simulink model "Batteri_Transducers_1I_1U"  (R2020b)
settings: Solver=VariableStepAuto  StartTime=0.0  StopTime=0.01  RelTol=1e-3
libraries: fl_lib x26, nesl_utility x10, ee_lib x2
settings Model: Creator=jenel  LastModifiedBy=jenel

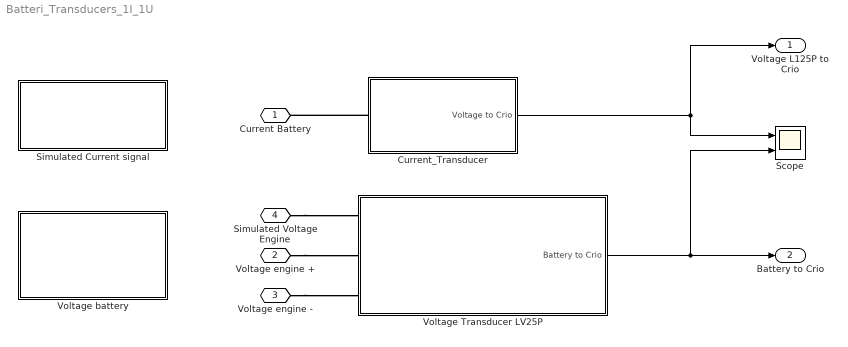
== system Batteri_Transducers_1I_1U ==
  Current_Transducer : Subsystem
  Scope : Scope  NumInputPorts=2
  Simulated Current signal : Subsystem
  Voltage Transducer LV25P : Subsystem
  Voltage battery : Subsystem
  Current Battery : PMIOPort  Side=Left
  Voltage engine + : PMIOPort  Port=2  Side=Left
  Voltage engine - : PMIOPort  Port=3  Side=Left
  Simulated Voltage Engine : PMIOPort  Port=4  Side=Right
  "Voltage L125P to Crio " : Outport
  Battery to Crio : Outport  Port=2
  wires:
  Voltage Transducer LV25P/1(Battery to Crio) -> Scope/2, Battery to Crio/1
  Current_Transducer/1(Voltage to Crio) -> Scope/1, "Voltage L125P to Crio "/1
  connections:
  Simulated Voltage Engine/RConn1 -- Voltage Transducer LV25P/LConn1
  Voltage engine +/RConn1 -- Voltage Transducer LV25P/LConn2
  Voltage engine -/RConn1 -- Voltage Transducer LV25P/LConn3
  Current_Transducer/LConn1 -- Current Battery/RConn1

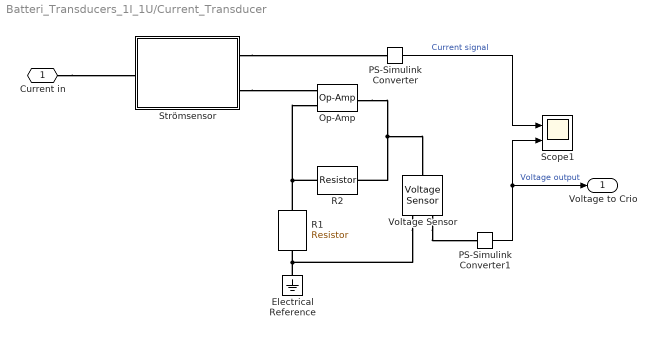
== system Batteri_Transducers_1I_1U/Current_Transducer ==
  Electrical Reference : fl_lib/Electrical/Electrical Elements/Electrical Reference
  Op-Amp : fl_lib/Electrical/Electrical Elements/Op-Amp  outI_specify=on  outI_priority=None  outI=0 A  outI_nominal_specify=off  outI_nominal_unit=A  outI_nominal_value=1
  PS-Simulink Converter : nesl_utility/PS-Simulink Converter  PhysicalDomain=network_engine_domain  SubClassName=ps_output  LeftPortType=input  RightPortType=output  PseudoPeriodic=off  Frequencies=[]  Unit=inherit  AffineConversion=off
  PS-Simulink Converter1 : nesl_utility/PS-Simulink Converter  PhysicalDomain=network_engine_domain  SubClassName=ps_output  LeftPortType=input  RightPortType=output  PseudoPeriodic=off  Frequencies=[]  Unit=inherit  AffineConversion=off
  R1 : fl_lib/Electrical/Electrical Elements/Resistor  R=1000 Ohm  i_specify=off  i_priority=None  i=0 A  i_nominal_specify=off  i_nominal_unit=A  i_nominal_value=1  v_specify=off  v_priority=None  v=0 V  v_nominal_specify=off  v_nominal_unit=V  v_nominal_value=1
  R2 : fl_lib/Electrical/Electrical Elements/Resistor  R=666.6667 Ohm  i_specify=off  i_priority=None  i=0 A  i_nominal_specify=off  i_nominal_unit=A  i_nominal_value=1  v_specify=off  v_priority=None  v=0 V  v_nominal_specify=off  v_nominal_unit=V  v_nominal_value=1
  Scope1 : Scope  NumInputPorts=2
  Strömsensor : Subsystem
  Voltage Sensor : fl_lib/Electrical/Electrical Sensors/Voltage Sensor
  Current in : PMIOPort  Side=Left
  Voltage to Crio : Outport
  wires:
  PS-Simulink Converter1/1 -> Scope1/2, Voltage to Crio/1  "Voltage output"
  PS-Simulink Converter/1 -> Scope1/1  "Current signal"
  connections:
  Strömsensor/RConn2 -- Op-Amp/LConn1
  R2/LConn1 -- R1/LConn1 -- Op-Amp/LConn2
  Current in/RConn1 -- Strömsensor/LConn1
  Strömsensor/RConn1 -- PS-Simulink Converter/LConn1
  Op-Amp/RConn1 -- Voltage Sensor/LConn1 -- R2/RConn1
  Electrical Reference/LConn1 -- R1/RConn1 -- Voltage Sensor/RConn2
  Voltage Sensor/RConn1 -- PS-Simulink Converter1/LConn1

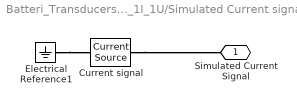
== system Batteri_Transducers_1I_1U/Simulated Current signal ==
  Current signal : ee_lib/Sources/Current Source  dc_current=200 mA  ac_current=0 mA  ac_shift=0 rad  ac_frequency=0 Hz  noise_mode=0  PSD=0 A^2/Hz  repeatability=1  auto_seed=153380492  user_seed=0  sample_time=1e-3 s  i_specify=off  i_priority=None  i=0 A  i_nominal_specify=off  i_nominal_unit=A  i_nominal_value=1  v_specify=off  v_priority=None  v=0 V  v_nominal_specify=off  v_nominal_unit=V  v_nominal_value=1
      settings: SourceProductBaseCode=PS
  Electrical Reference1 : fl_lib/Electrical/Electrical Elements/Electrical Reference
  Simulated Current Signal : PMIOPort  Side=Right
  connections:
  Electrical Reference1/LConn1 -- Current signal/RConn1
  Current signal/LConn1 -- Simulated Current Signal/RConn1

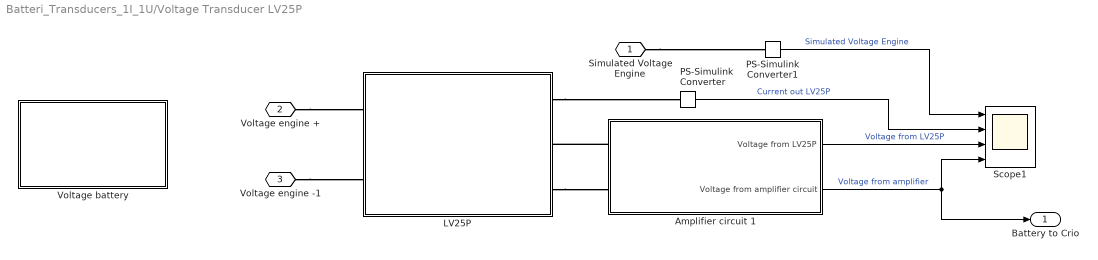
== system Batteri_Transducers_1I_1U/Voltage Transducer LV25P ==
  Amplifier circuit 1 : Subsystem
  LV25P : Subsystem
  PS-Simulink Converter : nesl_utility/PS-Simulink Converter  PhysicalDomain=network_engine_domain  SubClassName=ps_output  LeftPortType=input  RightPortType=output  PseudoPeriodic=off  Frequencies=[]  Unit=inherit  AffineConversion=off
  PS-Simulink Converter1 : nesl_utility/PS-Simulink Converter  PhysicalDomain=network_engine_domain  SubClassName=ps_output  LeftPortType=input  RightPortType=output  PseudoPeriodic=off  Frequencies=[]  Unit=inherit  AffineConversion=off
  Scope1 : Scope  NumInputPorts=4
  Voltage battery : Subsystem
  Simulated Voltage Engine : PMIOPort  Side=Left
  Voltage engine + : PMIOPort  Port=2  Side=Left
  Voltage engine -1 : PMIOPort  Port=3  Side=Left
  Battery to Crio : Outport
  wires:
  Amplifier circuit 1/1(Voltage from LV25P) -> Scope1/3  "Voltage from LV25P"
  PS-Simulink Converter1/1 -> Scope1/1  "Simulated Voltage Engine"
  Amplifier circuit 1/2(Voltage from amplifier circuit) -> Scope1/4, Battery to Crio/1  "Voltage from amplifier"
  PS-Simulink Converter/1 -> Scope1/2  "Current out LV25P"
  connections:
  Voltage engine +/RConn1 -- LV25P/LConn1
  Simulated Voltage Engine/RConn1 -- PS-Simulink Converter1/LConn1
  Amplifier circuit 1/LConn1 -- LV25P/RConn2
  LV25P/RConn1 -- PS-Simulink Converter/LConn1
  LV25P/RConn3 -- Amplifier circuit 1/LConn2
  Voltage engine -1/RConn1 -- LV25P/LConn2

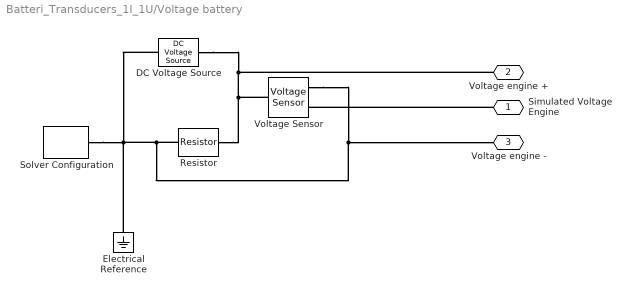
== system Batteri_Transducers_1I_1U/Voltage battery ==
  DC Voltage Source : ee_lib/Additional Components/SPICE Sources/DC Voltage Source  DC=144 V
  Electrical Reference : fl_lib/Electrical/Electrical Elements/Electrical Reference
  Resistor : fl_lib/Electrical/Electrical Elements/Resistor  R=10 Ohm  i_specify=off  i_priority=None  i=0 A  i_nominal_specify=off  i_nominal_unit=A  i_nominal_value=1  v_specify=off  v_priority=None  v=0 V  v_nominal_specify=off  v_nominal_unit=V  v_nominal_value=1
  Solver Configuration : nesl_utility/Solver Configuration  PhysicalDomain=network_engine_domain  SubClassName=solver  LeftPortType=input  RightPortType=generic  Tones=[]  Harmonics=[]  SimulateNoise=off  Profile=off  UseLocalSampling=off  EnableSwitchedLinearOptims=on  FrequencyDomain=off  UseCCode=off  RelTol=0.001  AbsTol=1e-06  MinStep=1e-09  ToWorkspace=off  RevertToSquareIcSolve=off  NumHomotopyIterations=100  PhasorMode=off  PhasorModeNumHarmonics=1  DoDC=off  ResidualTolerance=1e-09  UseLocalSolver=off  LocalSolverChoice=NE_BACKWARD_EULER_ADVANCER  LocalSolverSampleTime=0.001  DoFixedCost=off  MaxNonlinIter=3  MaxModeIter=2  ComputeImpulses=off  ImpulseIterations=2  LinearAlgebra=auto  EquationFormulation=NE_TIME_EF  DelaysMemoryBudget=1024  AutomaticFiltering=on  FilteringTimeConstant=0.001  PartitionStorageMethod=AS_NEEDED  PartitionMemoryBudget=1024  PartitionMethod=ROBUST
  Voltage Sensor : fl_lib/Electrical/Electrical Sensors/Voltage Sensor
  Simulated Voltage Engine : PMIOPort  Side=Right
  Voltage engine + : PMIOPort  Port=2  Side=Right
  Voltage engine - : PMIOPort  Port=3  Side=Right
  connections:
  Simulated Voltage Engine/RConn1 -- Voltage Sensor/RConn1
  Voltage Sensor/LConn1 -- DC Voltage Source/LConn1 -- Voltage engine +/RConn1 -- Resistor/RConn1
  Resistor/LConn1 -- Voltage Sensor/RConn2 -- Voltage engine -/RConn1 -- DC Voltage Source/RConn1 -- Electrical Reference/LConn1 -- Solver Configuration/RConn1

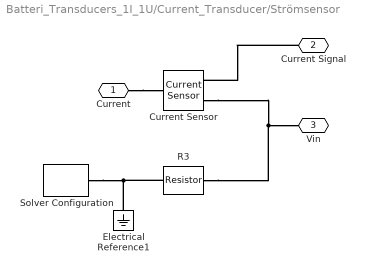
== system Batteri_Transducers_1I_1U/Current_Transducer/Strömsensor ==
  Current Sensor : fl_lib/Electrical/Electrical Sensors/Current Sensor
  Electrical Reference1 : fl_lib/Electrical/Electrical Elements/Electrical Reference
  R3 : fl_lib/Electrical/Electrical Elements/Resistor  R=30 Ohm  i_specify=off  i_priority=None  i=0 A  i_nominal_specify=off  i_nominal_unit=A  i_nominal_value=1  v_specify=off  v_priority=None  v=0 V  v_nominal_specify=off  v_nominal_unit=V  v_nominal_value=1
  Solver Configuration : nesl_utility/Solver Configuration  PhysicalDomain=network_engine_domain  SubClassName=solver  LeftPortType=input  RightPortType=generic  Tones=[]  Harmonics=[]  SimulateNoise=off  Profile=off  UseLocalSampling=off  EnableSwitchedLinearOptims=on  FrequencyDomain=off  UseCCode=off  RelTol=0.001  AbsTol=1e-06  MinStep=1e-09  ToWorkspace=off  RevertToSquareIcSolve=off  NumHomotopyIterations=100  PhasorMode=off  PhasorModeNumHarmonics=1  DoDC=off  ResidualTolerance=1e-09  UseLocalSolver=off  LocalSolverChoice=NE_BACKWARD_EULER_ADVANCER  LocalSolverSampleTime=0.001  DoFixedCost=off  MaxNonlinIter=3  MaxModeIter=2  ComputeImpulses=off  ImpulseIterations=2  LinearAlgebra=auto  EquationFormulation=NE_TIME_EF  DelaysMemoryBudget=1024  AutomaticFiltering=on  FilteringTimeConstant=0.001  PartitionStorageMethod=AS_NEEDED  PartitionMemoryBudget=1024  PartitionMethod=ROBUST
  Current : PMIOPort  Side=Left
  Current Signal : PMIOPort  Port=2  Side=Right
  Vin : PMIOPort  Port=3  Side=Right
  connections:
  Current/RConn1 -- Current Sensor/LConn1
  Current Signal/RConn1 -- Current Sensor/RConn1
  Current Sensor/RConn2 -- Vin/RConn1 -- R3/LConn1
  Electrical Reference1/LConn1 -- Solver Configuration/RConn1 -- R3/RConn1

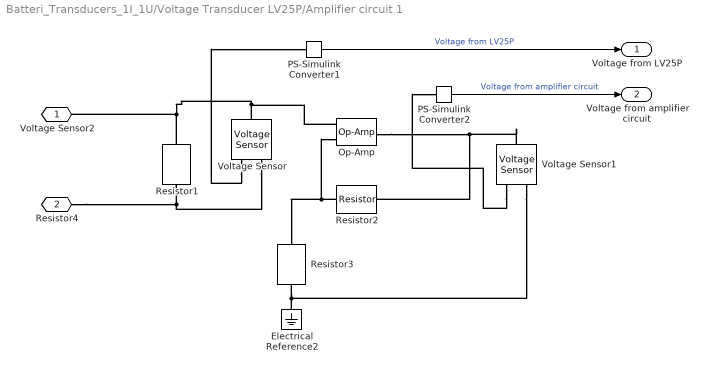
== system Batteri_Transducers_1I_1U/Voltage Transducer LV25P/Amplifier circuit 1 ==
  Electrical Reference2 : fl_lib/Electrical/Electrical Elements/Electrical Reference
  Op-Amp : fl_lib/Electrical/Electrical Elements/Op-Amp  outI_specify=off  outI_priority=None  outI=0 A  outI_nominal_specify=off  outI_nominal_unit=A  outI_nominal_value=1
  PS-Simulink Converter1 : nesl_utility/PS-Simulink Converter  PhysicalDomain=network_engine_domain  SubClassName=ps_output  LeftPortType=input  RightPortType=output  PseudoPeriodic=off  Frequencies=[]  Unit=inherit  AffineConversion=off
  PS-Simulink Converter2 : nesl_utility/PS-Simulink Converter  PhysicalDomain=network_engine_domain  SubClassName=ps_output  LeftPortType=input  RightPortType=output  PseudoPeriodic=off  Frequencies=[]  Unit=inherit  AffineConversion=off
  Resistor1 : fl_lib/Electrical/Electrical Elements/Resistor  R=100 Ohm  i_specify=off  i_priority=None  i=0 A  i_nominal_specify=off  i_nominal_unit=A  i_nominal_value=1  v_specify=off  v_priority=None  v=0 V  v_nominal_specify=off  v_nominal_unit=V  v_nominal_value=1
  Resistor2 : fl_lib/Electrical/Electrical Elements/Resistor  R=30 kOhm  i_specify=off  i_priority=None  i=0 A  i_nominal_specify=off  i_nominal_unit=A  i_nominal_value=1  v_specify=off  v_priority=None  v=0 V  v_nominal_specify=off  v_nominal_unit=V  v_nominal_value=1
  Resistor3 : fl_lib/Electrical/Electrical Elements/Resistor  R=10 kOhm  i_specify=off  i_priority=None  i=0 A  i_nominal_specify=off  i_nominal_unit=A  i_nominal_value=1  v_specify=off  v_priority=None  v=0 V  v_nominal_specify=off  v_nominal_unit=V  v_nominal_value=1
  Voltage Sensor : fl_lib/Electrical/Electrical Sensors/Voltage Sensor
  Voltage Sensor1 : fl_lib/Electrical/Electrical Sensors/Voltage Sensor
  Voltage Sensor2 : PMIOPort  Side=Left
  Resistor4 : PMIOPort  Port=2  Side=Left
  Voltage from LV25P : Outport
  Voltage from amplifier circuit : Outport  Port=2
  wires:
  PS-Simulink Converter2/1 -> Voltage from amplifier circuit/1  "Voltage from amplifier circuit"
  PS-Simulink Converter1/1 -> Voltage from LV25P/1  "Voltage from LV25P"
  connections:
  Resistor1/LConn1 -- Op-Amp/LConn1 -- Voltage Sensor/LConn1 -- Voltage Sensor2/RConn1
  Op-Amp/RConn1 -- Voltage Sensor1/LConn1 -- Resistor2/RConn1
  Voltage Sensor/RConn2 -- Resistor4/RConn1 -- Resistor1/RConn1
  Voltage Sensor1/RConn1 -- PS-Simulink Converter2/LConn1
  Electrical Reference2/LConn1 -- Voltage Sensor1/RConn2 -- Resistor3/RConn1
  Resistor2/LConn1 -- Op-Amp/LConn2 -- Resistor3/LConn1
  Voltage Sensor/RConn1 -- PS-Simulink Converter1/LConn1

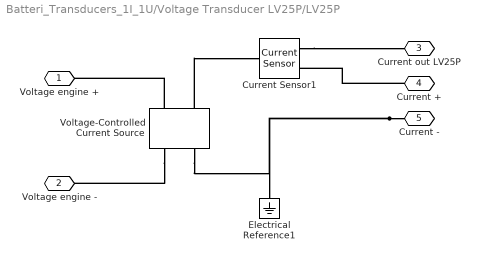
== system Batteri_Transducers_1I_1U/Voltage Transducer LV25P/LV25P ==
  Current Sensor1 : fl_lib/Electrical/Electrical Sensors/Current Sensor
  Electrical Reference1 : fl_lib/Electrical/Electrical Elements/Electrical Reference
  Voltage-Controlled Current Source : fl_lib/Electrical/Electrical Sources/Voltage-Controlled Current Source  K=0.000125 1/Ohm  v1_specify=off  v1_priority=None  v1=0 V  v1_nominal_specify=off  v1_nominal_unit=V  v1_nominal_value=1  i2_specify=off  i2_priority=None  i2=0 A  i2_nominal_specify=off  i2_nominal_unit=A  i2_nominal_value=1
      settings: SourceProductBaseCode=SS  InternalSimscapePortConfiguration="{\"Bottom\":[],\"Left\":[{\"id\":\"p1\",\"label\":\"+\",\"type\":\"foundation.electrical.electrical\"},{\"id\":\"head\",\"label\":\"\",\"type\":\"foundation.electrical.electrical\"}],\"Right\":[{\"id\":\"n1\",\"label\":\"-\",\"type\":\"foundation.electrical.electrical\"},{\"id\":\"tail\",\"label\":\"\",\"type\":\"foundation.electrical.electrical\"}],\"Top\":[]}"
  Voltage engine + : PMIOPort  Side=Left
  Voltage engine - : PMIOPort  Port=2  Side=Left
  Current out LV25P : PMIOPort  Port=3  Side=Right
  Current + : PMIOPort  Port=4  Side=Right
  Current - : PMIOPort  Port=5  Side=Right
  connections:
  Current -/RConn1 -- Voltage-Controlled Current Source/RConn2 -- Electrical Reference1/LConn1
  Voltage-Controlled Current Source/LConn2 -- Current Sensor1/LConn1
  Current +/RConn1 -- Current Sensor1/RConn2
  Voltage-Controlled Current Source/RConn1 -- Voltage engine -/RConn1
  Current Sensor1/RConn1 -- Current out LV25P/RConn1
  Voltage-Controlled Current Source/LConn1 -- Voltage engine +/RConn1

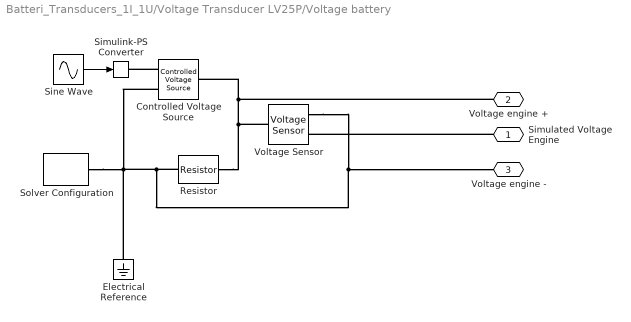
== system Batteri_Transducers_1I_1U/Voltage Transducer LV25P/Voltage battery ==
  Controlled Voltage Source : fl_lib/Electrical/Electrical Sources/Controlled Voltage Source
  Electrical Reference : fl_lib/Electrical/Electrical Elements/Electrical Reference
  Resistor : fl_lib/Electrical/Electrical Elements/Resistor  R=10 Ohm  i_specify=off  i_priority=None  i=0 A  i_nominal_specify=off  i_nominal_unit=A  i_nominal_value=1  v_specify=off  v_priority=None  v=0 V  v_nominal_specify=off  v_nominal_unit=V  v_nominal_value=1
  Simulink-PS Converter : nesl_utility/Simulink-PS Converter  PhysicalDomain=network_engine_domain  SubClassName=ps_input  LeftPortType=input  RightPortType=output  PseudoPeriodic=off  Frequencies=[]  NoiseDistribution=none  NoiseParameters=[]  Unit=1  AffineConversion=off  FilteringAndDerivatives=provide  SimscapeFilterOrder=1  InputFilterTimeConstant=0.001  UdotUserProvided=0
  Sine Wave : Sin  Amplitude=200  Frequency=200  SampleTime=0
  Solver Configuration : nesl_utility/Solver Configuration  PhysicalDomain=network_engine_domain  SubClassName=solver  LeftPortType=input  RightPortType=generic  Tones=[]  Harmonics=[]  SimulateNoise=off  Profile=off  UseLocalSampling=off  EnableSwitchedLinearOptims=on  FrequencyDomain=off  UseCCode=off  RelTol=0.001  AbsTol=1e-06  MinStep=1e-09  ToWorkspace=off  RevertToSquareIcSolve=off  NumHomotopyIterations=100  PhasorMode=off  PhasorModeNumHarmonics=1  DoDC=off  ResidualTolerance=1e-09  UseLocalSolver=off  LocalSolverChoice=NE_BACKWARD_EULER_ADVANCER  LocalSolverSampleTime=0.001  DoFixedCost=off  MaxNonlinIter=3  MaxModeIter=2  ComputeImpulses=off  ImpulseIterations=2  LinearAlgebra=auto  EquationFormulation=NE_TIME_EF  DelaysMemoryBudget=1024  AutomaticFiltering=on  FilteringTimeConstant=0.001  PartitionStorageMethod=AS_NEEDED  PartitionMemoryBudget=1024  PartitionMethod=ROBUST
  Voltage Sensor : fl_lib/Electrical/Electrical Sensors/Voltage Sensor
  Simulated Voltage Engine : PMIOPort  Side=Right
  Voltage engine + : PMIOPort  Port=2  Side=Right
  Voltage engine - : PMIOPort  Port=3  Side=Right
  wires:
  Sine Wave/1 -> Simulink-PS Converter/1
  connections:
  Controlled Voltage Source/RConn1 -- Simulink-PS Converter/RConn1
  Simulated Voltage Engine/RConn1 -- Voltage Sensor/RConn1
  Voltage Sensor/LConn1 -- Controlled Voltage Source/LConn1 -- Voltage engine +/RConn1 -- Resistor/RConn1
  Resistor/LConn1 -- Voltage Sensor/RConn2 -- Voltage engine -/RConn1 -- Electrical Reference/LConn1 -- Solver Configuration/RConn1 -- Controlled Voltage Source/RConn2
